simulink model "task2"  (R2018b)
settings: Solver=VariableStepAuto  StartTime=0.0  StopTime=20  RelTol=1e-3
values from neighbouring files (symbols this model uses):
  Dq0 = zeros(3,1)    [task2_full.m]
  Kd = [[ 4,   0,  0];       [ 0,   6,  0];       [ 0,   0,  6]]    [task2_full.m]
  Kp = [[ 3, 0,  0];       [ 0, 6,  0];       [ 0, 0,  4]]    [task2_full.m]
  q0 = zeros(3,1)    [task2_full.m]
settings Model: Creator=Magne Sirnes  LastModifiedBy=Magne Sirnes

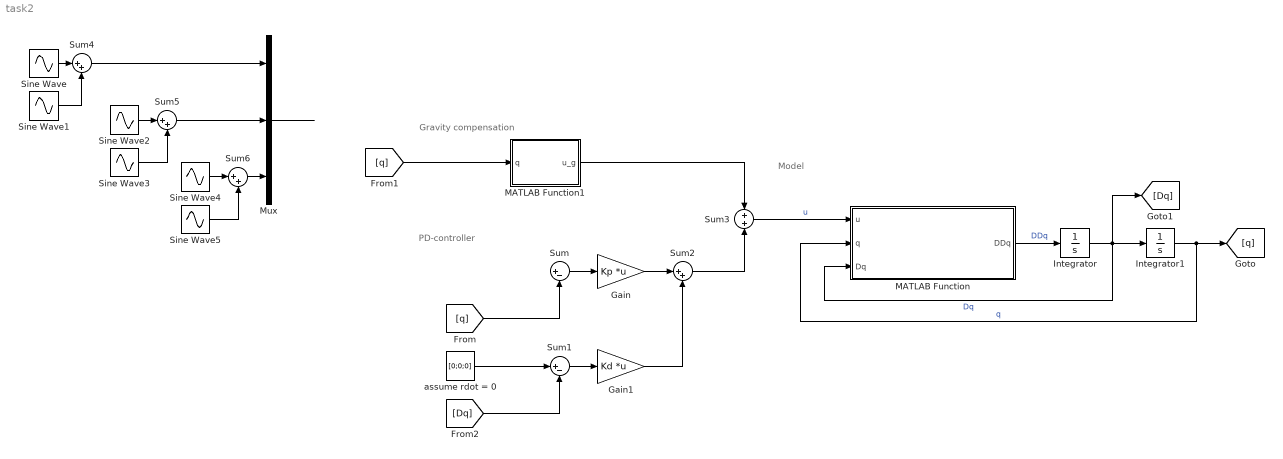
== system task2 ==
  note: Gravity compensation
  note: PD-controller
  note: Model
  Gain : Gain  Gain=Kp  Multiplication=Matrix(K*u)
  Gain1 : Gain  Gain=Kd  Multiplication=Matrix(K*u)
  Integrator : Integrator  InitialCondition=Dq0
  Integrator1 : Integrator  InitialCondition=q0
  MATLAB Function : MATLAB Function  TreatAsAtomicUnit=on
  MATLAB Function1 : MATLAB Function  TreatAsAtomicUnit=on
  Mux : Mux  Inputs=3
  Sine Wave : Sin  Frequency=0.05  SampleTime=0
  Sine Wave1 : Sin  Amplitude=0.2  Frequency=0.2  SampleTime=0
  Sine Wave2 : Sin  Amplitude=0.5  Frequency=0.05  SampleTime=0
  Sine Wave3 : Sin  Amplitude=0.1  Frequency=0.1  SampleTime=0
  Sine Wave4 : Sin  Amplitude=-1  Frequency=0.05  SampleTime=0
  Sine Wave5 : Sin  Amplitude=0.1  Frequency=0.1  SampleTime=0
  Sum : Sum  Inputs=|+-
  Sum1 : Sum  Inputs=|+-
  Sum{2,4..6} (4 alike) : Sum  Inputs=|++
  Sum3 : Sum  Inputs=+|+
  assume rdot = 0 : Constant  Value=[0;0;0]
  wires:
  MATLAB Function/1(DDq) -> Integrator/1  "DDq"
  Integrator/1 -> Integrator1/1, [Dq], MATLAB Function/3(Dq)  "Dq"
  Integrator1/1 -> [q], MATLAB Function/2(q)  "q"
  ? -> Sum/1  "r"
  [q] -> Sum/2
  [Dq] -> Sum1/2
  assume rdot = 0/1 -> Sum1/1
  Sum/1 -> Gain/1
  Gain/1 -> Sum2/1
  Sum1/1 -> Gain1/1
  Gain1/1 -> Sum2/2
  Sum2/1 -> Sum3/2
  MATLAB Function1/1(u_g) -> Sum3/1
  Sum3/1 -> MATLAB Function/1(u)  "u"
  [q] -> MATLAB Function1/1(q)
  Sine Wave/1 -> Sum4/1
  Sine Wave1/1 -> Sum4/2
  Sum4/1 -> Mux/1
  Sine Wave2/1 -> Sum5/1
  Sine Wave3/1 -> Sum5/2
  Sum5/1 -> Mux/2
  Sine Wave5/1 -> Sum6/2
  Sine Wave4/1 -> Sum6/1
  Sum6/1 -> Mux/3
  Mux/1 -> ?

== matlab function task2/MATLAB Function1 ==
  data: q input; u_g output
function u_g = gravity_comp(q)

q1 = q(1); q2 = q(2); q3 = q(3);

% snippet from provided script
m1  = 5;      m2 = 5;       m3 = 5;
lc1 = 0.5/2; lc2 = -0.5/2; lc3 = 0.5/2;
gy    = 9.81;
G = [(m3 * cos(q1 + q3) * lc3 + sin(q1) * q2 * m2 + sin(q1) * q2 * m3 + sin(q1) * lc1 * m1 - sin(q1) * m2 * lc2) * gy; -(m2 + m3) * cos(q1) * gy; m3 * cos(q1 + q3) * lc3 * gy;];
% snippet end

u_g = G;

== matlab function task2/MATLAB Function ==
  data: u input; q input; Dq input; DDq output
function DDq = matrix_model(u, q, Dq)

q1  = q(1);   q2 = q(2);   q3 = q(3);
dq1 = Dq(1); dq2 = Dq(2); dq3 = Dq(3);

% snippet from provided script
m1  = 5;      m2 = 5;       m3 = 5;
l1  = 0.5;    l2 = 0.5;     l3 = 0.5;
lc1 = 0.5/2; lc2 = -0.5/2; lc3 = 0.5/2;
In1yy = 1/12*(m1*(l1)^2);
In2zz = 1/12*(m2*(l2)^2);
In3zz = 1/12*(m3*(l3)^2);
gy    = 9.81;
G = [(m3 * cos(q1 + q3) * lc3 + sin(q1) * q2 * m2 + sin(q1) * q2 * m3 + sin(q1) * lc1 * m1 - sin(q1) * m2 * lc2) * gy; -(m2 + m3) * cos(q1) * gy; m3 * cos(q1 + q3) * lc3 * gy;];
C = [(-0.2e1 * m3 * lc3 * cos(q1) * sin(q1 + q3) + 0.2e1 * m3 * lc3 * sin(q1) * cos(q1 + q3) + 0.2e1 * (m2 + m3) * q2 - 0.2e1 * m2 * lc2) * dq2 / 0.2e1 + (-0.2e1 * m3 * lc3 * cos(q1) * q2 * cos(q1 + q3) - 0.2e1 * m3 * lc3 * sin(q1) * q2 * sin(q1 + q3)) * dq3 / 0.2e1 (-0.2e1 * m3 * lc3 * cos(q1) * sin(q1 + q3) + 0.2e1 * m3 * lc3 * sin(q1) * cos(q1 + q3) + 0.2e1 * (m2 + m3) * q2 - 0.2e1 * m2 * lc2) * dq1 / 0.2e1 (-0.2e1 * m3 * lc3 * cos(q1) * q2 * cos(q1 + q3) - 0.2e1 * m3 * lc3 * sin(q1) * q2 * sin(q1 + q3)) * dq1 / 0.2e1 + (-m3 * lc3 * cos(q1) * q2 * cos(q1 + q3) - m3 * lc3 * sin(q1) * q2 * sin(q1 + q3)) * dq3; (-m3 * lc3 * sin(q1) * cos(q1 + q3) + m3 * lc3 * cos(q1) * sin(q1 + q3) - (m2 + m3) * q2 + m2 * lc2) * dq1 + (-0.2e1 * m3 * lc3 * sin(q1) * cos(q1 + q3) + 0.2e1 * m3 * lc3 * cos(q1) * sin(q1 + q3)) * dq3 / 0.2e1 0 (-0.2e1 * m3 * lc3 * sin(q1) * cos(q1 + q3) + 0.2e1 * m3 * lc3 * cos(q1) * sin(q1 + q3)) * dq1 / 0.2e1 + (-m3 * lc3 * sin(q1) * cos(q1 + q3) + m3 * lc3 * cos(q1) * sin(q1 + q3)) * dq3; (m3 * lc3 * cos(q1) * q2 * cos(q1 + q3) + m3 * lc3 * sin(q1) * q2 * sin(q1 + q3)) * dq1 + (0.2e1 * m3 * lc3 * sin(q1) * cos(q1 + q3) - 0.2e1 * m3 * lc3 * cos(q1) * sin(q1 + q3)) * dq2 / 0.2e1 (0.2e1 * m3 * lc3 * sin(q1) * cos(q1 + q3) - 0.2e1 * m3 * lc3 * cos(q1) * sin(q1 + q3)) * dq1 / 0.2e1 0;];
D = [0.2e1 * m3 * lc3 * cos(q1 + q3) * sin(q1) * q2 - 0.2e1 * m3 * lc3 * sin(q1 + q3) * cos(q1) * q2 + (m2 + m3) * q2 ^ 2 - 0.2e1 * m2 * lc2 * q2 + m1 * lc1 ^ 2 + In1yy + m2 * lc2 ^ 2 + In3zz + In2zz + m3 * lc3 ^ 2 -m3 * lc3 * sin(q1) * sin(q1 + q3) - m3 * lc3 * cos(q1) * cos(q1 + q3) m3 * lc3 ^ 2 - m3 * lc3 * sin(q1 + q3) * cos(q1) * q2 + m3 * lc3 * cos(q1 + q3) * sin(q1) * q2 + In3zz; -m3 * lc3 * sin(q1) * sin(q1 + q3) - m3 * lc3 * cos(q1) * cos(q1 + q3) m2 + m3 -m3 * lc3 * sin(q1) * sin(q1 + q3) - m3 * lc3 * cos(q1) * cos(q1 + q3); m3 * lc3 ^ 2 - m3 * lc3 * sin(q1 + q3) * cos(q1) * q2 + m3 * lc3 * cos(q1 + q3) * sin(q1) * q2 + In3zz -m3 * lc3 * sin(q1) * sin(q1 + q3) - m3 * lc3 * cos(q1) * cos(q1 + q3) m3 * lc3 ^ 2 + In3zz;];
% snippet end

DDq = D\( u - C*Dq - G);
